simulink model "system_2022 [23-03-03]"  (R2022a)
settings: Solver=FixedStepAuto  StartTime=0.0  StopTime=30  FixedStep=0.05  MinStep=0.01  RelTol=1e-3  EnableMultiTasking=on
libraries: mbedblockslib x24, simulink x6, hdlsllib x6, slpidlib x3
(part 2 of 3)

== system system_2022 [23-03-03]/Subsystem/Pressure_Sensor_1/Pressure Conversion ==
  note: psi -> cmH2O
  note: Inspiration Pressure Calculation
      | Pg3 - Honeywell SPI Comms
  note: hex -> psi
  y : Inport
  Add : Sum
  Constant : Constant  Value=1638
  Constant1 : Constant  Value=120
  Constant2 : Constant  Value=13107
  Constant3 : Constant  Value=-60
  Constant4 : Constant  Value=1.01972
  Display : Display
  Display1 : Display
      settings: Format=hex (Stored Integer)
  Divide : Product  Inputs=*/
  Product : Product
  Product1 : Product
  Subtract : Sum  Inputs=+-
  Pressure : Outport
  wires:
  Constant/1 -> Subtract/2
  Subtract/1 -> Product/2
  Constant1/1 -> Product/1
  Product/1 -> Divide/1
  Constant2/1 -> Divide/2
  Constant3/1 -> Add/2
  Divide/1 -> Add/1
  Add/1 -> Product1/1
  Constant4/1 -> Product1/2
  Product1/1 -> Pressure/1, Display/1
  y/1 -> Display1/1, Subtract/1

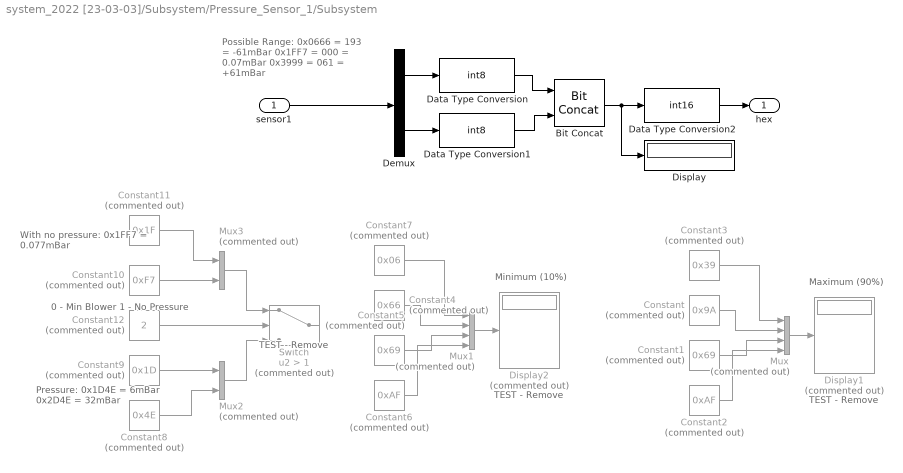
== system system_2022 [23-03-03]/Subsystem/Pressure_Sensor_1/Subsystem ==
  note: TEST - Remove
  note: 0 - Min Blower
      | 1 - No Pressure
  note: With no pressure:
      | 0x1FF7 = 0.077mBar
  note: Maximum (90%)
  note: Minimum (10%)
  note: Possible Range:
      | 0x0666 = 193 = -61mBar
      | 0x1FF7 = 000 = 0.07mBar
      | 0x3999 = 061 = +61mBar
  note: Pressure:
      | 0x1D4E = 6mBar
      | 0x2D4E = 32mBar
  note: TEST - Remove
  note: TEST - Remove
  sensor1 : Inport
  Bit Concat : hdlsllib/Logic and Bit Operations/Bit Concat  numInputs=2
  Constant : Constant  Commented=on  Value=0x9A
  Constant1 : Constant  Commented=on  Value=0x69
  Constant10 : Constant  Commented=on  Value=0xF7
  Constant11 : Constant  Commented=on  Value=0x1F
  Constant12 : Constant  Commented=on  Value=2
  Constant2 : Constant  Commented=on  Value=0xAF
  Constant3 : Constant  Commented=on  Value=0x39
  Constant4 : Constant  Commented=on  Value=0x66
  Constant5 : Constant  Commented=on  Value=0x69
  Constant6 : Constant  Commented=on  Value=0xAF
  Constant7 : Constant  Commented=on  Value=0x06
  Constant8 : Constant  Commented=on  Value=0x4E
  Constant9 : Constant  Commented=on  Value=0x1D
  Data Type Conversion : DataTypeConversion  OutDataTypeStr=int8  SaturateOnIntegerOverflow=off  RndMeth=Floor
  Data Type Conversion1 : DataTypeConversion  OutDataTypeStr=int8  SaturateOnIntegerOverflow=off  RndMeth=Floor
  Data Type Conversion2 : DataTypeConversion  OutDataTypeStr=int16  SaturateOnIntegerOverflow=off  RndMeth=Floor
  Demux : Demux  Outputs=2
  Display : Display
      settings: Format=hex (Stored Integer)
  Display1 : Display  Commented=on
      settings: Format=hex (Stored Integer)
  Display2 : Display  Commented=on
      settings: Format=hex (Stored Integer)
  Mux : Mux  Commented=on
  Mux1 : Mux  Commented=on
  Mux2 : Mux  Commented=on  Inputs=2
  Mux3 : Mux  Commented=on  Inputs=2
  Switch : Switch  Commented=on  Criteria=u2 > Threshold  Threshold=1  SaturateOnIntegerOverflow=off  InputSameDT=off
  hex : Outport
  wires:
  Constant3/1 -> Mux/1
  Constant/1 -> Mux/2
  Constant1/1 -> Mux/3
  Constant2/1 -> Mux/4
  Data Type Conversion/1 -> Bit Concat/1
  Data Type Conversion1/1 -> Bit Concat/2
  Demux/1 -> Data Type Conversion/1
  Demux/2 -> Data Type Conversion1/1
  Bit Concat/1 -> Display/1, Data Type Conversion2/1
  Mux/1 -> Display1/1
  Mux1/1 -> Display2/1
  Constant7/1 -> Mux1/1
  Constant6/1 -> Mux1/4
  Constant5/1 -> Mux1/3
  Constant4/1 -> Mux1/2
  Constant9/1 -> Mux2/1
  Constant8/1 -> Mux2/2
  Constant10/1 -> Mux3/2
  Constant11/1 -> Mux3/1
  Constant12/1 -> Switch/2
  Mux3/1 -> Switch/1
  Mux2/1 -> Switch/3
  Data Type Conversion2/1 -> hex/1
  sensor1/1 -> Demux/1

== system system_2022 [23-03-03]/Subsystem/Pressure_Sensor_1/Subsystem2 ==
  note: Need Global Array??
  note: Update single element of input array
  note: Extract Elements
  Array : Inport
  Index1 : Inport  Port=2
  Sense1 : Inport  Port=3
  Assignment : Assignment  IndexMode=Zero-based  DiagnosticForDimensions=Warning  IndexOptions=Index vector (port)  Indices=0  OutputSizes=1
  Out1 : Outport
  tag scope: PRES_AR1=global
  wires:
  Index1/1 -> Assignment/3
  Sense1/1 -> Assignment/2
  Assignment/1 -> [PRES_AR1], Out1/1
  Array/1 -> Assignment/1

== system system_2022 [23-03-03]/Subsystem/Pressure_Sensor_2/Pressure Conversion ==
  note: psi -> cmH2O
  note: Inspiration Pressure Calculation
      | Pg3 - Honeywell SPI Comms
  note: hex -> psi
  y : Inport
  Add : Sum
  Constant : Constant  Value=1638
  Constant1 : Constant  Value=120
  Constant2 : Constant  Value=13107
  Constant3 : Constant  Value=-60
  Constant4 : Constant  Value=1.01972
  Display : Display
  Display1 : Display
      settings: Format=hex (Stored Integer)
  Divide : Product  Inputs=*/
  Product : Product
  Product1 : Product
  Subtract : Sum  Inputs=+-
  Pressure : Outport
  wires:
  Constant/1 -> Subtract/2
  Subtract/1 -> Product/2
  Constant1/1 -> Product/1
  Product/1 -> Divide/1
  Constant2/1 -> Divide/2
  Constant3/1 -> Add/2
  Divide/1 -> Add/1
  Add/1 -> Product1/1
  Constant4/1 -> Product1/2
  Product1/1 -> Pressure/1, Display/1
  y/1 -> Display1/1, Subtract/1

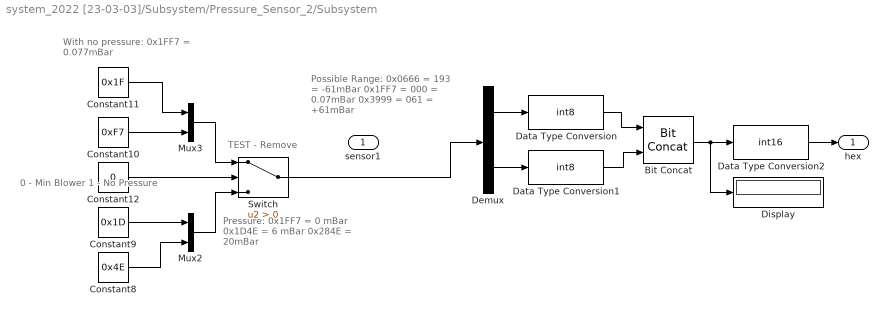
== system system_2022 [23-03-03]/Subsystem/Pressure_Sensor_2/Subsystem ==
  note: 0 - Min Blower
      | 1 - No Pressure
  note: With no pressure:
      | 0x1FF7 = 0.077mBar
  note: Possible Range:
      | 0x0666 = 193 = -61mBar
      | 0x1FF7 = 000 = 0.07mBar
      | 0x3999 = 061 = +61mBar
  note: Pressure:
      | 0x1FF7 = 0 mBar
      | 0x1D4E = 6 mBar
      | 0x284E = 20mBar
  note: TEST - Remove
  sensor1 : Inport
  Bit Concat : hdlsllib/Logic and Bit Operations/Bit Concat  numInputs=2
  Constant10 : Constant  Value=0xF7
  Constant11 : Constant  Value=0x1F
  Constant12 : Constant  Value=0
  Constant8 : Constant  Value=0x4E
  Constant9 : Constant  Value=0x1D
  Data Type Conversion : DataTypeConversion  OutDataTypeStr=int8  SaturateOnIntegerOverflow=off  RndMeth=Floor
  Data Type Conversion1 : DataTypeConversion  OutDataTypeStr=int8  SaturateOnIntegerOverflow=off  RndMeth=Floor
  Data Type Conversion2 : DataTypeConversion  OutDataTypeStr=int16  SaturateOnIntegerOverflow=off  RndMeth=Floor
  Demux : Demux  Outputs=2
  Display : Display
      settings: Format=hex (Stored Integer)
  Mux2 : Mux  Inputs=2
  Mux3 : Mux  Inputs=2
  Switch : Switch  Criteria=u2 > Threshold  SaturateOnIntegerOverflow=off  InputSameDT=off
  hex : Outport
  wires:
  Data Type Conversion/1 -> Bit Concat/1
  Data Type Conversion1/1 -> Bit Concat/2
  Demux/1 -> Data Type Conversion/1
  Demux/2 -> Data Type Conversion1/1
  Bit Concat/1 -> Display/1, Data Type Conversion2/1
  Constant9/1 -> Mux2/1
  Constant8/1 -> Mux2/2
  Constant10/1 -> Mux3/2
  Constant11/1 -> Mux3/1
  Constant12/1 -> Switch/2
  Mux3/1 -> Switch/1
  Mux2/1 -> Switch/3
  Switch/1 -> Demux/1
  Data Type Conversion2/1 -> hex/1

== system system_2022 [23-03-03]/Subsystem/Pressure_Sensor_2/Subsystem2 ==
  note: Update single element of input array
  note: Array "GoTo"
  Index1 : Inport
  Sense1 : Inport  Port=2
  Array : Inport  Port=3
  Assignment : Assignment  IndexMode=Zero-based  DiagnosticForDimensions=Warning  IndexOptions=Index vector (port)  Indices=0  OutputSizes=1
  Flow2 : Outport
  tag scope: PRES_AR2=global
  wires:
  Index1/1 -> Assignment/3
  Sense1/1 -> Assignment/2
  Assignment/1 -> [PRES_AR2], Flow2/1
  Array/1 -> Assignment/1

== system system_2022 [23-03-03]/Subsystem/Sensor_Monitor/Flow1_Monitor ==
  note: Exhale Flow Rate 1
      | Create Sub-System Status Commands
      | While inside threshold - Normal opertation (forward flow value)
      | If above/below threshold - Triggers alarm (alert value + alrm_trg)
  note: Alarm is triggered if Flow Rate is: [5 < Flow1 > 25] (SLM)
  note: Flow1 Trigger Values:
      | 0x41 = 65 - Normal Op
      | 0x42 = 66 - FlowRate2 High
      | 0x43 = 67 - FlowRate2 Low
  Flow1 : Inport
  Hi_Alert1 : Subsystem  TreatAsAtomicUnit=on
  If : If  IfExpression=(u1 <= 10)  ElseIfExpressions=(u1 >= 80)
  Lo_Alert1 : Subsystem  TreatAsAtomicUnit=on
  Merge : Merge  Inputs=3
  No_Alert1 : Subsystem  TreatAsAtomicUnit=on
  Fl1_Alrm : Outport
  wires:
  Flow1/1 -> If/1
  If/3 -> No_Alert1/Action
  No_Alert1/1(no_v) -> Merge/3
  Hi_Alert1/1(Out1) -> Merge/2
  Lo_Alert1/1(Out1) -> Merge/1
  If/2 -> Hi_Alert1/Action
  If/1 -> Lo_Alert1/Action
  Merge/1 -> Fl1_Alrm/1

== system system_2022 [23-03-03]/Subsystem/Sensor_Monitor/Flow2_Monitor ==
  note: Exhale Flow Rate 2
      | Create Sub-System Status Commands
      | While inside threshold - Normal opertation (forward flow value)
      | If above/below threshold - Triggers alarm (alert value + alrm_trg)
  note: Alarm is triggered if Flow Rate is: [5 < Flow1 > 25] (SLM)
  note: Flow1 Trigger Values:
      | 0x41 = 65 - Normal Op
      | 0x42 = 66 - FlowRate2 High
      | 0x43 = 67 - FlowRate2 Low
  Flow2 : Inport
  Hi_Alert2 : Subsystem  TreatAsAtomicUnit=on
  If : If  IfExpression=(u1 <= 10)  ElseIfExpressions=(u1 >= 80)
  Lo_Alert2 : Subsystem  TreatAsAtomicUnit=on
  Merge : Merge  Inputs=3
  No_Alert2 : Subsystem  TreatAsAtomicUnit=on
  Fl2_Alrm : Outport
  wires:
  Flow2/1 -> If/1
  If/3 -> No_Alert2/Action
  No_Alert2/1(no_v) -> Merge/3
  Hi_Alert2/1(Out1) -> Merge/2
  Lo_Alert2/1(Out1) -> Merge/1
  If/2 -> Hi_Alert2/Action
  If/1 -> Lo_Alert2/Action
  Merge/1 -> Fl2_Alrm/1

== system system_2022 [23-03-03]/Subsystem/Sensor_Monitor/Pressure1_Monitor ==
  note: Alarm is triggered if Pressure is: [5 < Prs > 25] (cmH20)
      | But Blower should also adjust pressure according to sensor reading.
  note: (Ex_Pressure)
      | Create Sub-System Status Commands
      | While inside threshold - Normal opertation (forward pressure value)
      | If above/below threshold - Triggers alarm (alert value + alrm_trg)
  Pr_I1 : Inport
  Display : Display
  Hi_Alert1 : Subsystem  TreatAsAtomicUnit=on
  If : If  IfExpression=(u1 <= 5)  ElseIfExpressions=(u1 >= 20)
  Lo_Alert1 : Subsystem  TreatAsAtomicUnit=on
  Merge : Merge  Inputs=3
  No_Alert1 : Subsystem  TreatAsAtomicUnit=on
  Pr1_Alrm : Outport
  wires:
  If/1 -> Lo_Alert1/Action
  If/3 -> No_Alert1/Action
  If/2 -> Hi_Alert1/Action
  Pr_I1/1 -> Display/1, If/1
  No_Alert1/1(no_v) -> Merge/3
  Lo_Alert1/1(Out1) -> Merge/1
  Hi_Alert1/1(Out1) -> Merge/2
  Merge/1 -> Pr1_Alrm/1

== system system_2022 [23-03-03]/Subsystem/Sensor_Monitor/Pressure2_Monitor ==
  note: Alarm is triggered if Pressure is: [5 < Prs > 25] (cmH20)
      | But Blower should also adjust pressure according to sensor reading.
  note: (Ex_Pressure)
      | Create Sub-System Status Commands
      | While inside threshold - Normal opertation (forward pressure value)
      | If above/below threshold - Triggers alarm (alert value + alrm_trg)
  Pr_E2 : Inport
  Display : Display
  Hi_Alert1 : Subsystem  TreatAsAtomicUnit=on
  If : If  IfExpression=(u1 <= 5)  ElseIfExpressions=(u1 >= 20)
  Lo_Alert1 : Subsystem  TreatAsAtomicUnit=on
  Merge : Merge  Inputs=3
  No_Alert1 : Subsystem  TreatAsAtomicUnit=on
  Pr2_Alrm : Outport
  wires:
  If/1 -> Lo_Alert1/Action
  If/3 -> No_Alert1/Action
  If/2 -> Hi_Alert1/Action
  Pr_E2/1 -> Display/1, If/1
  No_Alert1/1(no_v) -> Merge/3
  Lo_Alert1/1(Out1) -> Merge/1
  Hi_Alert1/1(Out1) -> Merge/2
  Merge/1 -> Pr2_Alrm/1

== system system_2022 [23-03-03]/Subsystem/Sensor_Monitor/Subsystem ==
  note: Alarm Hierarchy & Output
      | (Merge Sensor Alerts to single output)
  note: SIMULTANEOUS ALERTS?
      | -> Will Alert from Highest Priority
  note: Flow1_Alert
  note: Pres1_Alert
  note: Only 1 Alert Out
  note: Normal Value:
      | 0x31 (49) - Pressure1
      | 0x41 (65) - Flow1
      | 0x51 (81) - Pressure2
      | 0x61 (97) - Flow2
      | 0x71 (113) - FiO2
  note: Pres2_Alert
  note: Flow2_Alert
  note: FiO2_Alert
  note: ALARM Responses:
      | 0x21 - Normal Operation
      | 0x22 - Alarm Time_Out (2min)
      | 0x23 - Others ?
  Pr1_Alrm : Inport
  Fl1_Alrm : Inport  Port=2
  Pr2_Alrm : Inport  Port=3
  Fl2_Alrm : Inport  Port=4
  Fi_Alrm : Inport  Port=5
  FiO2_Alert : Subsystem  TreatAsAtomicUnit=on
  Flow_Alert1 : Subsystem  TreatAsAtomicUnit=on
  Flow_Alert2 : Subsystem  TreatAsAtomicUnit=on
  If : If  NumInputs=5  IfExpression=(u1 >= 50)  ElseIfExpressions=(u2 >= 66), (u3 >= 82), (u4 >= 98), (u5 >= 114)  ZeroCross=off
  Merge : Merge  Inputs=6
  No_Alert : Subsystem  TreatAsAtomicUnit=on
  Press_Alert1 : Subsystem  TreatAsAtomicUnit=on
  Press_Alert2 : Subsystem  TreatAsAtomicUnit=on
  ALRM_Out : Outport
  wires:
  If/6 -> No_Alert/Action
  Merge/1 -> ALRM_Out/1
  Pr2_Alrm/1 -> Press_Alert2/1(P2_Alrm), If/3
  Fl2_Alrm/1 -> Flow_Alert2/1(F2_Alrm), If/4
  Fi_Alrm/1 -> FiO2_Alert/1(FiO2_Alrm), If/5
  If/3 -> Press_Alert2/Action
  If/4 -> Flow_Alert2/Action
  If/5 -> FiO2_Alert/Action
  Press_Alert2/1(Out1) -> Merge/3
  Flow_Alert2/1(Out1) -> Merge/4
  FiO2_Alert/1(Out1) -> Merge/5
  No_Alert/1(Out1) -> Merge/6
  Fl1_Alrm/1 -> Flow_Alert1/1(F1_Alrm), If/2
  Pr1_Alrm/1 -> Press_Alert1/1(P1_Alrm), If/1
  If/2 -> Flow_Alert1/Action
  If/1 -> Press_Alert1/Action
  Flow_Alert1/1(Out1) -> Merge/2
  Press_Alert1/1(Out1) -> Merge/1

== system system_2022 [23-03-03]/Subsystem/Sub-Systems Read/HMI_Test_Input ==
  Dummy Startup : Stateflow chart  TreatAsAtomicUnit=on
  HMI Graph Test : Stateflow chart  TreatAsAtomicUnit=on
  Reshape : Reshape  OutputDimensionality=Column vector (2-D)
  H_Cmd : Outport
  wires:
  Reshape/1 -> H_Cmd/1
  HMI Graph Test/1(output) -> Reshape/1

== system system_2022 [23-03-03]/Subsystem/Sub-Systems Write/Combine All ==
  note: 51 = 0x33 = No Alarm
      | 33 = 0x21 = No Alarm
  note: Select highest priority Alert & Update to HMI Array
  note: Write 5 byte array to HMI
      | + 1 Alarm byte
  note: Output Highest Priority
      | 1st - SubSystem
      | 2nd - Sensors
  HMI : Inport
  AlmSBS : Inport  Port=2
  AlmSNS : Inport  Port=3
  Constant2 : Constant  Value=5
  Display : Display
  Display1 : Display
  Display2 : Display
  Hi_Alert1 : Subsystem  TreatAsAtomicUnit=on
  Hi_Alert2 : Subsystem  TreatAsAtomicUnit=on
  If : If  NumInputs=2  IfExpression=(u1 > 33)  ElseIfExpressions=(u2 >= 20)
  Lo_Alert1 : Subsystem  TreatAsAtomicUnit=on
  Merge : Merge  Inputs=3
  Subsystem3 : Subsystem
  Alarm : Outport
  HMI_Array : Outport  Port=2
  wires:
  HMI/1 -> Subsystem3/3(Array)
  Constant2/1 -> Subsystem3/1(Index1)
  Subsystem3/1(Flow2) -> HMI_Array/1
  If/2 -> Hi_Alert1/Action
  If/1 -> Lo_Alert1/Action
  AlmSBS/1 -> Display/1, Lo_Alert1/1(AlmSBS), If/1
  AlmSNS/1 -> Display1/1, Hi_Alert1/1(AlmSNS), If/2
  Hi_Alert1/1(Out1) -> Merge/2
  Lo_Alert1/1(Out1) -> Merge/1
  Merge/1 -> Subsystem3/2(Sense1), Display2/1, Alarm/1
  If/3 -> Hi_Alert2/Action
  Hi_Alert2/1(Out1) -> Merge/3

== system system_2022 [23-03-03]/Subsystem/System Update and Heirarchy/Alarm Priority ==
  note: Create final ALARM message
  note: What if BOTH ? - consecutive
  note: Single byte Alert:
      | UPPER 4-bits:
      | 0x10 - Power
      | 0x20 - Alarm
      | 0x30 - Pressure
      | 0x40 - Flow...
      |
      | LOWER 4-bits:
      | over/under/bat_%/time_out
  note: Remove this whole block and forward Alarm Codes directly
  note: Alarm Alerts:
      | 0x21 - No Alarm
      | 0x22 - Over_Time
  note: PSU Alerts:
      | 0x11 - Normal (AC)
      | 0x12 - Battery 75%
      | 0x13 - Battery 50%
      | 0x14 - Battery 25%
  P_Alrm : Inport
  A_Alrm : Inport  Port=2
  Alarm Alert : Subsystem  TreatAsAtomicUnit=on
  Data Type Conversion : DataTypeConversion  OutDataTypeStr=double  SaturateOnIntegerOverflow=off  RndMeth=Floor
  Display2 : Display
  If : If  NumInputs=2  IfExpression=(u1 > 17)  ElseIfExpressions=(u2 > 33)
  Merge : Merge  Inputs=3
  No_Alarm1 : Subsystem  TreatAsAtomicUnit=on
  Power Alert : Subsystem  TreatAsAtomicUnit=on
  ALRM_Out : Outport
  wires:
  P_Alrm/1 -> Data Type Conversion/1, If/1
  A_Alrm/1 -> If/2
  If/1 -> Power Alert/Action
  Merge/1 -> Display2/1, ALRM_Out/1
  Power Alert/1(Out1) -> Merge/1
  Alarm Alert/1(Out1) -> Merge/2
  No_Alarm1/1(Out1) -> Merge/3
  Data Type Conversion/1 -> Power Alert/1(P_Alrm)
  If/2 -> Alarm Alert/Action
  If/3 -> No_Alarm1/Action

== system system_2022 [23-03-03]/Subsystem/System Update and Heirarchy/Get Value and Array Index ==
  note: Get byte[0]
  note: Extract Specific Byte from HMI_Input Array
  note: Get byte[1]
  Usr_In : Inport
  Constant1 : Constant  OutDataTypeStr=uint8
  Constant2 : Constant  Value=0  OutDataTypeStr=uint8
  Display1 : Display
  Display12 : Display
  Display4 : Display
  Index Vector : MultiPortSwitch  DataPortOrder=Zero-based contiguous  Inputs=1  zeroidx=on  OutDataTypeStr=uint8  SaturateOnIntegerOverflow=off  InputSameDT=off
  Index Vector1 : MultiPortSwitch  DataPortOrder=Zero-based contiguous  Inputs=1  zeroidx=on  OutDataTypeStr=uint8  SaturateOnIntegerOverflow=off  InputSameDT=off
  HMI_Cmd1 : Outport
  New_Val1 : Outport  Port=2
  wires:
  Index Vector/1 -> HMI_Cmd1/1, Display4/1
  Constant2/1 -> Index Vector/1
  Usr_In/1 -> Display12/1, Index Vector1/2, Index Vector/2
  Constant1/1 -> Index Vector1/1
  Index Vector1/1 -> Display1/1, New_Val1/1

== system system_2022 [23-03-03]/Subsystem/System Update and Heirarchy/Initial IPAP EPAP ==
  note: [1x2] to [2x1]
  note: Initial IPAP & EPAP Values:
      | (only on boot-up)
  H_Cmd : Inport
  Chart : Stateflow chart  TreatAsAtomicUnit=on
      settings: PortSchema="{\"entries\":[{\"content\":{\"sides\":[{\"content\":{\"connectorIds\":[]},\"type\":\"ConnectorPlacement.EquallySpacedRectSide\",\"uuid\":\"6628deca-e0b8-40ca-949f-ac0e837bdfd6\"},{\"content\":{\"connectorIds\":[\"Out2\",\"Out1\"],\"side\":\"RIGHT\"},\"type\":\"ConnectorPlacement.EquallySpacedRectSide\",\"uuid\":\"942c872d-7aee-48e1-8ef8-861eef53b55a\"},{\"content\":{\"connectorIds\":[],\"side\":\"TOP\"},\"type\":\"ConnectorPlacement.EquallySpacedRectSide\",\"uuid\":\"7d4bff24-2b40-487e-be4f-fa01986134b0\"}]},\"type\":\"ConnectorPlacement.EquallySpacedConnector\",\"uuid\":\"61848f08-0c78-4d83-a956-79c751d6cd3c\"}],\"packageUris\":[\"http://schema.mathworks.com/mf0/Connector/R2020b\"],\"version\":\"1.0\"}"
  Display : Display
  If : If  IfExpression=u1 > 4
  If Action Subsystem : Subsystem  TreatAsAtomicUnit=on
  If Action Subsystem1 : Subsystem  TreatAsAtomicUnit=on
  Merge : Merge
  Reshape : Reshape  OutputDimensionality=Column vector (2-D)
  output : Outport
  wires:
  Merge/1 -> Display/1, output/1
  If Action Subsystem1/1(Out1) -> Merge/2
  If/1 -> If Action Subsystem1/Action
  If/2 -> If Action Subsystem/Action
  Chart/2(nope) -> If/1
  H_Cmd/1 -> If Action Subsystem1/1(output)
  If Action Subsystem/1(Out1) -> Merge/1
  Chart/1(output) -> Reshape/1
  Reshape/1 -> If Action Subsystem/1(output)

== system system_2022 [23-03-03]/Subsystem/System Update and Heirarchy/Power_CMD ==
  note: REMOVED PSU CHECK (ALARM & HMI WILL CHECK)
  note: PASS PSU CODE DIRECTLY
  note: 0x14 = 20dec
  note: (PSU)
      | Read Sub-System Status Commands
      | Normal operation = No 2nd byte
      | Event trigger (2) = DC voltage forwarded
  note: Get Lower 4 bits
  note: Battery Status:
      | 0x10 - AC
      | 0x11 - 75%
      | 0x12 - 50%
      | 0x13 - 25%
  note: PSU Alerts:
      | 0x11 - Normal (AC)
      | 0x12 - Battery 75%
      | 0x13 - Battery 50%
      | 0x14 - Battery 25%
  note: Error Code (99)
  P_Cmd : Inport
  AC POWER : Subsystem  Commented=on  TreatAsAtomicUnit=on
  Bitwise Operator1 : simulink/Logic and Bit Operations/Bitwise Operator  Commented=on  logicop=AND  UseBitMask=on  BitMask=bin2dec('00001111')  BitMaskRealWorld=Stored Integer
  Constant : Constant  Commented=on  Value=0x13
  Constant2 : Constant  Commented=on  Value=0x14  SampleTime=-1
  Constant3 : Constant  Commented=on  Value=0x63  SampleTime=-1
  DC POWER : Subsystem  Commented=on  TreatAsAtomicUnit=on
  Display1 : Display  Commented=on
      settings: Format=hex (Stored Integer)
  ERROR MSG1 : Subsystem  Commented=on  TreatAsAtomicUnit=on
  Merge1 : Merge  Commented=on  Inputs=4
  Power_Other : Subsystem  Commented=on  TreatAsAtomicUnit=on
  Switch Case1 : SwitchCase  Commented=on  CaseConditions={0x01, 0x02, 0x03}
  P_Alrm : Outport
  wires:
  Switch Case1/4 -> ERROR MSG1/Action
  Constant2/1 -> Power_Other/1(In1)
  Switch Case1/1 -> AC POWER/Action
  Switch Case1/3 -> Power_Other/Action
  Bitwise Operator1/1 -> Switch Case1/1
  Switch Case1/2 -> DC POWER/Action
  Constant3/1 -> ERROR MSG1/1(In1)
  Power_Other/1(Out1) -> Merge1/3
  ERROR MSG1/1(Out1) -> Merge1/4
  AC POWER/1(Out1) -> Merge1/1
  DC POWER/1(DC_out) -> Merge1/2
  P_Cmd/1 -> P_Alrm/1
  Constant/1 -> DC POWER/1(DC_in), Bitwise Operator1/1
  Merge1/1 -> Display1/1

== system system_2022 [23-03-03]/Subsystem/System Update and Heirarchy/Update Internal Variables ==
  note: Remove Var_Arr:
      | Unless used internally?
  note: Update the system variable with User_Input
      | Save new value to correct Array element for system update
  note: Variables:
      | [0] - CPAP
      | [1] - EPAP
      | [2] - IPAP
      | [3] - FiO2
      | [4] - APNEA
      | [5] - Mode
  note: Array Element
  note: Value to be stored
  note: Should be from updated HMI
      | Input Value Array[0-4] .
      | Single value at the moment.
  note: HMI - INPUTS:
      | 0x03 (03) - CPAP
      | 0x13 (19) - EPAP
      | 0x23 (35) - IPAP
      | 0x33 (51) - FiO2
      | 0x43 (67) - APNEA
  note: Other Inputs:
      | 0x11 (17) - Start
      | 0x19 (25) - Mode
  HMI_Cmd1 : Inport
  New_Val1 : Inport  Port=2
  Display : Display
  Display1 : Display
  Display2 : Display
  Get_HMI_Values : Subsystem
  HMI_CMD1 : Subsystem
  wires:
  HMI_CMD1/1(Element1) -> Get_HMI_Values/1(Element1), Display/1
  HMI_Cmd1/1 -> HMI_CMD1/1(H_Cmd)
  Get_HMI_Values/1(Var_Arr) -> Display2/1
  New_Val1/1 -> Get_HMI_Values/2(Value1), Display1/1

== system system_2022 [23-03-03]/Subsystem/Sensor_Monitor/Flow1_Monitor/Hi_Alert1 ==
  note: If within normal pressure range,
      | forward that value to HMI for display
  note: Above FlowRate threshold = 0x42
  note: 0x42 = 66 dec
  note: Above Flow Rate (1) Threshold
  Action Port : ActionPort  ActionPortLabel=elseif((u1 >= 80))
  Alert1 : Constant  Value=66
  Out1 : Outport
  wires:
  Alert1/1 -> Out1/1

== system system_2022 [23-03-03]/Subsystem/Sensor_Monitor/Flow1_Monitor/Lo_Alert1 ==
  note: Below Flow Rate (1) Threshold
  note: Below FlowRate Threshold = 0x43
  note: 0x43 = 67 dec
  Action Port : ActionPort  ActionPortLabel=if((u1 <= 10))
  Alert1 : Constant  Value=67
  Out1 : Outport
  wires:
  Alert1/1 -> Out1/1

== system system_2022 [23-03-03]/Subsystem/Sensor_Monitor/Flow1_Monitor/No_Alert1 ==
  note: No Alert (normal range) = 0x01
  note: 0x41 = 65 dec
  note: Within Flow Rate (1) Threshold
  Action Port : ActionPort  ActionPortLabel=else
  Alert1 : Constant  Value=65
  no_v : Outport
  wires:
  Alert1/1 -> no_v/1

== system system_2022 [23-03-03]/Subsystem/Sensor_Monitor/Flow2_Monitor/Hi_Alert2 ==
  note: If within normal pressure range,
      | forward that value to HMI for display
  note: Above FlowRate threshold = 0x42
  note: 0x62 = 98 dec
  note: Below Flow Rate (2) Threshold
  Action Port : ActionPort  ActionPortLabel=elseif((u1 >= 80))
  Alert1 : Constant  Value=98
  Out1 : Outport
  wires:
  Alert1/1 -> Out1/1

== system system_2022 [23-03-03]/Subsystem/Sensor_Monitor/Flow2_Monitor/Lo_Alert2 ==
  note: Below Flow Rate (2) Threshold
  note: Below FlowRate Threshold = 0x43
  note: 0x63 = 99 dec
  Action Port : ActionPort  ActionPortLabel=if((u1 <= 10))
  Alert1 : Constant  Value=99
  Out1 : Outport
  wires:
  Alert1/1 -> Out1/1

== system system_2022 [23-03-03]/Subsystem/Sensor_Monitor/Flow2_Monitor/No_Alert2 ==
  note: No Alert (normal range) = 0x01
  note: 0x61 = 97 dec
  note: Within Flow Rate (2) Threshold
  Action Port : ActionPort  ActionPortLabel=else
  Alert1 : Constant  Value=97
  no_v : Outport
  wires:
  Alert1/1 -> no_v/1

== system system_2022 [23-03-03]/Subsystem/Sensor_Monitor/Pressure1_Monitor/Hi_Alert1 ==
  note: Above Pressure threshold
  note: 0x32 = 50 dec
  note: Above Pressure Threshold = 0x32
  Action Port : ActionPort  ActionPortLabel=elseif((u1 >= 20))
  Alert1 : Constant  Value=50
  Out1 : Outport
  wires:
  Alert1/1 -> Out1/1

== system system_2022 [23-03-03]/Subsystem/Sensor_Monitor/Pressure1_Monitor/Lo_Alert1 ==
  note: 0x33 = 51 dec
  note: Below Pressure Threshold = 0x33
  Action Port : ActionPort  ActionPortLabel=if((u1 <= 5))
  Alert1 : Constant  Value=51
  Out1 : Outport
  wires:
  Alert1/1 -> Out1/1

== system system_2022 [23-03-03]/Subsystem/Sensor_Monitor/Pressure1_Monitor/No_Alert1 ==
  note: No Trigger - Within Range
  note: No Alert (normal range)
  note: If within normal pressure range,
      | forward that value to HMI for display
  note: 0x31 - 49 dec
  Action Port : ActionPort  ActionPortLabel=else
  Alert1 : Constant  Value=49
  no_v : Outport
  wires:
  Alert1/1 -> no_v/1

== system system_2022 [23-03-03]/Subsystem/Sensor_Monitor/Pressure2_Monitor/Hi_Alert1 ==
  note: Above Pressure threshold
  note: 0x52 = 82 dec
  note: Above Pressure (2) Threshold = 0x52
  Action Port : ActionPort  ActionPortLabel=elseif((u1 >= 20))
  Alert1 : Constant  Value=82
  Out1 : Outport
  wires:
  Alert1/1 -> Out1/1

== system system_2022 [23-03-03]/Subsystem/Sensor_Monitor/Pressure2_Monitor/Lo_Alert1 ==
  note: 0x53 = 83 dec
  note: Below Pressure (2) Threshold = 0x53
  Action Port : ActionPort  ActionPortLabel=if((u1 <= 5))
  Alert1 : Constant  Value=83
  Out1 : Outport
  wires:
  Alert1/1 -> Out1/1

== system system_2022 [23-03-03]/Subsystem/Sensor_Monitor/Pressure2_Monitor/No_Alert1 ==
  note: No Trigger - Within Range
  note: No Alert (normal range)
  note: If within normal pressure range,
      | forward that value to HMI for display
  note: 0x31 - 49 dec
  Action Port : ActionPort  ActionPortLabel=else
  Alert1 : Constant  Value=49
  no_v : Outport
  wires:
  Alert1/1 -> no_v/1

== system system_2022 [23-03-03]/Subsystem/Sensor_Monitor/Subsystem/FiO2_Alert ==
  note: Pressure Alert
  FiO2_Alrm : Inport
  Action Port : ActionPort  ActionPortLabel=elseif( (u5 >= 114))
  Out1 : Outport
  wires:
  FiO2_Alrm/1 -> Out1/1

== system system_2022 [23-03-03]/Subsystem/Sensor_Monitor/Subsystem/Flow_Alert1 ==
  note: Either Pressure OR Power Alert!
  F1_Alrm : Inport
  Action Port : ActionPort  ActionPortLabel=elseif((u2 >= 66))
  Out1 : Outport
  wires:
  F1_Alrm/1 -> Out1/1

== system system_2022 [23-03-03]/Subsystem/Sensor_Monitor/Subsystem/Flow_Alert2 ==
  note: Pressure Alert
  F2_Alrm : Inport
  Action Port : ActionPort  ActionPortLabel=elseif( (u4 >= 98))
  Out1 : Outport
  wires:
  F2_Alrm/1 -> Out1/1

== system system_2022 [23-03-03]/Subsystem/Sensor_Monitor/Subsystem/No_Alert ==
  note: 0X01 = NO ALERTS
  note: Normal Opertaion (No Alerts)
  Action Port : ActionPort  ActionPortLabel=else
  Constant : Constant  Value=33
  Out1 : Outport
  wires:
  Constant/1 -> Out1/1

== system system_2022 [23-03-03]/Subsystem/Sensor_Monitor/Subsystem/Press_Alert1 ==
  note: Pressure Alert
  P1_Alrm : Inport
  Action Port : ActionPort  ActionPortLabel=if((u1 >= 50))
  Out1 : Outport
  wires:
  P1_Alrm/1 -> Out1/1

== system system_2022 [23-03-03]/Subsystem/Sensor_Monitor/Subsystem/Press_Alert2 ==
  note: Pressure (2) High or Low
  P2_Alrm : Inport
  Action Port : ActionPort  ActionPortLabel=elseif( (u3 >= 82))
  Out1 : Outport
  wires:
  P2_Alrm/1 -> Out1/1

== system system_2022 [23-03-03]/Subsystem/Sub-Systems Write/Combine All/Hi_Alert1 ==
  note: Sensor Alerts Take Lowest Priority
  AlmSNS : Inport
  Action Port : ActionPort  ActionPortLabel=elseif((u2 >= 20))
  Out1 : Outport
  wires:
  AlmSNS/1 -> Out1/1

== system system_2022 [23-03-03]/Subsystem/Sub-Systems Write/Combine All/Hi_Alert2 ==
  note: 0x21 = 33 dec
  note: If No Alert
  Action Port : ActionPort  ActionPortLabel=else
  No Alert1 : Constant  Value=33
  Out1 : Outport
  wires:
  No Alert1/1 -> Out1/1

== system system_2022 [23-03-03]/Subsystem/Sub-Systems Write/Combine All/Lo_Alert1 ==
  note: Sub-System Alert Take Highest Priority
  AlmSBS : Inport
  Action Port : ActionPort  ActionPortLabel=if((u1 > 33))
  Out1 : Outport
  wires:
  AlmSBS/1 -> Out1/1

== system system_2022 [23-03-03]/Subsystem/Sub-Systems Write/Combine All/Subsystem3 ==
  note: Need Global Array??
  note: Update single element of input array
  Index1 : Inport
  Sense1 : Inport  Port=2
  Array : Inport  Port=3
  Assignment : Assignment  IndexMode=Zero-based  DiagnosticForDimensions=Warning  IndexOptions=Index vector (port)  Indices=0  OutputSizes=1
  Flow2 : Outport
  wires:
  Index1/1 -> Assignment/3
  Sense1/1 -> Assignment/2
  Assignment/1 -> Flow2/1
  Array/1 -> Assignment/1

== system system_2022 [23-03-03]/Subsystem/System Update and Heirarchy/Alarm Priority/Alarm Alert ==
  note: 0x22 = 34 dec
  note: ALARM OVER 2 MINUTES
  Action Port : ActionPort  ActionPortLabel=elseif((u2 > 33))
  Constant : Constant  Value=34
  Out1 : Outport
  wires:
  Constant/1 -> Out1/1

== system system_2022 [23-03-03]/Subsystem/System Update and Heirarchy/Alarm Priority/No_Alarm1 ==
  note: 0x11 = Normal Operation
  note: Normal Opertaion (No Alerts)
  Action Port : ActionPort  ActionPortLabel=else
  Constant : Constant  Value=33
  Out1 : Outport
  wires:
  Constant/1 -> Out1/1

== system system_2022 [23-03-03]/Subsystem/System Update and Heirarchy/Alarm Priority/Power Alert ==
  note: Battery Alert & Capacity in same byte
  note: PSU Power Alert + Battery %
  P_Alrm : Inport
  Action Port : ActionPort  ActionPortLabel=if((u1 > 17))
  Out1 : Outport
  wires:
  P_Alrm/1 -> Out1/1

== system system_2022 [23-03-03]/Subsystem/System Update and Heirarchy/Initial IPAP EPAP/If Action Subsystem ==
  output : Inport
  Action Port : ActionPort  ActionPortLabel=else
  Out1 : Outport
  wires:
  output/1 -> Out1/1

== system system_2022 [23-03-03]/Subsystem/System Update and Heirarchy/Initial IPAP EPAP/If Action Subsystem1 ==
  output : Inport
  Action Port : ActionPort  ActionPortLabel=if(u1 > 4)
  Out1 : Outport
  wires:
  output/1 -> Out1/1

== system system_2022 [23-03-03]/Subsystem/System Update and Heirarchy/Power_CMD/AC POWER ==
  Action Port : ActionPort
  Constant : Constant  Value=0x10
  Out1 : Outport
  wires:
  Constant/1 -> Out1/1

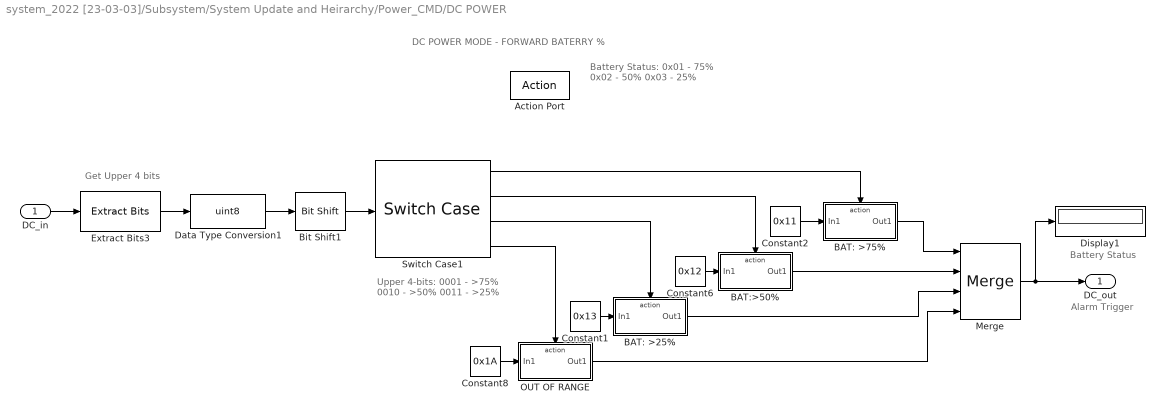
== system system_2022 [23-03-03]/Subsystem/System Update and Heirarchy/Power_CMD/DC POWER ==
  note: Battery Status
  note: Upper 4-bits:
      | 0001 - >75%
      | 0010 - >50%
      | 0011 - >25%
  note: DC POWER MODE - FORWARD BATERRY %
  note: Get Upper 4 bits
  note: Alarm Trigger
  note: Battery Status:
      | 0x01 - 75%
      | 0x02 - 50%
      | 0x03 - 25%
  DC_in : Inport
  Action Port : ActionPort
  BAT: >25% : Subsystem  TreatAsAtomicUnit=on
  BAT: >75% : Subsystem  TreatAsAtomicUnit=on
  BAT:>50% : Subsystem  TreatAsAtomicUnit=on
  Bit Shift1 : hdlsllib/Logic and Bit Operations/Bit Shift  mode=Shift Right Logical  N=4
  Constant1 : Constant  Value=0x13  SampleTime=-1
  Constant2 : Constant  Value=0x11  SampleTime=-1
  Constant6 : Constant  Value=0x12  SampleTime=-1
  Constant8 : Constant  Value=0x1A  SampleTime=-1
  Data Type Conversion1 : DataTypeConversion  OutDataTypeStr=uint8  SaturateOnIntegerOverflow=off  RndMeth=Floor
  Display1 : Display
      settings: Format=hex (Stored Integer)
  Extract Bits3 : simulink/Logic and Bit Operations/Extract Bits  bitsToExtract=Upper half  numBits=8  bitIdxRange=[0 7]  outScalingMode=Preserve fixed-point scaling
  Merge : Merge  Inputs=4
  OUT OF RANGE : Subsystem  TreatAsAtomicUnit=on
  Switch Case1 : SwitchCase  CaseConditions={0x01, 0x02, 0x03}
  DC_out : Outport
  wires:
  Switch Case1/3 -> BAT: >25%/Action
  Merge/1 -> DC_out/1, Display1/1
  Constant8/1 -> OUT OF RANGE/1(In1)
  OUT OF RANGE/1(Out1) -> Merge/4
  BAT: >75%/1(Out1) -> Merge/1
  Extract Bits3/1 -> Data Type Conversion1/1
  Switch Case1/2 -> BAT:>50%/Action
  Bit Shift1/1 -> Switch Case1/1
  BAT:>50%/1(Out1) -> Merge/2
  Constant6/1 -> BAT:>50%/1(In1)
  Data Type Conversion1/1 -> Bit Shift1/1
  BAT: >25%/1(Out1) -> Merge/3
  Switch Case1/4 -> OUT OF RANGE/Action
  Switch Case1/1 -> BAT: >75%/Action
  Constant2/1 -> BAT: >75%/1(In1)
  Constant1/1 -> BAT: >25%/1(In1)
  DC_in/1 -> Extract Bits3/1

== system system_2022 [23-03-03]/Subsystem/System Update and Heirarchy/Power_CMD/ERROR MSG1 ==
  In1 : Inport
  Action Port : ActionPort
  Out1 : Outport
  wires:
  In1/1 -> Out1/1

== system system_2022 [23-03-03]/Subsystem/System Update and Heirarchy/Power_CMD/Power_Other ==
  note: Do what with each
      | Triggerd bit?
  In1 : Inport
  Action Port : ActionPort
  Out1 : Outport
  wires:
  In1/1 -> Out1/1

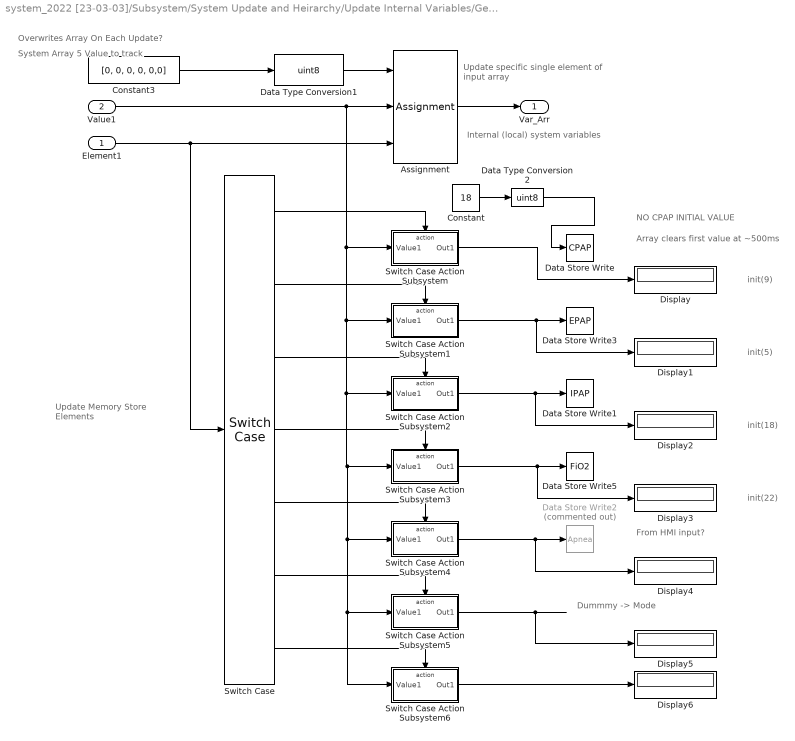
== system system_2022 [23-03-03]/Subsystem/System Update and Heirarchy/Update Internal Variables/Get_HMI_Values ==
  note: init(18)
  note: NO CPAP INITIAL VALUE
  note: Internal (local) system variables
  note: System Array
      | 5 Value to track
  note: Update specific single
      | element of input array
  note: Overwrites Array On Each Update?
  note: Update Memory
      | Store Elements
  note: From HMI input?
  note: init(5)
  note: init(9)
  note: init(22)
  note: Array clears first value at ~500ms
  note: Dummmy -> Mode
  Element1 : Inport
  Value1 : Inport  Port=2
  Assignment : Assignment  IndexMode=Zero-based  DiagnosticForDimensions=Warning  IndexOptions=Index vector (port)  Indices=0  OutputSizes=1
  Constant : Constant  Value=18
  Constant3 : Constant  Value=[0, 0, 0, 0, 0,0]
  Data Store Write : DataStoreWrite  DataStoreName=CPAP  IndexOptions=Index vector (dialog)  Indices=1  OutputSizes=1
  Data Store Write1 : DataStoreWrite  DataStoreName=IPAP  DataStoreElements=IPAP  IndexOptions=Index vector (dialog)  Indices=1  OutputSizes=1
  Data Store Write2 : DataStoreWrite  Commented=on  DataStoreName=Apnea  IndexOptions=Index vector (dialog)  Indices=1  OutputSizes=1
  Data Store Write3 : DataStoreWrite  DataStoreName=EPAP  DataStoreElements=EPAP  IndexOptions=Index vector (dialog)  Indices=1  OutputSizes=1
  Data Store Write5 : DataStoreWrite  DataStoreName=FiO2  IndexOptions=Index vector (dialog)  Indices=1  OutputSizes=1
  Data Type Conversion1 : DataTypeConversion  OutDataTypeStr=uint8  SaturateOnIntegerOverflow=off  RndMeth=Floor
  Data Type Conversion2 : DataTypeConversion  OutDataTypeStr=uint8  SaturateOnIntegerOverflow=off  RndMeth=Floor
  Display{,1..6} (7 alike) : Display
  Switch Case : SwitchCase  CaseConditions={0,1,2,3,4,5}
  Switch Case Action Subsystem : Subsystem  TreatAsAtomicUnit=on
  Switch Case Action Subsystem1 : Subsystem  TreatAsAtomicUnit=on
  Switch Case Action Subsystem2 : Subsystem  TreatAsAtomicUnit=on
  Switch Case Action Subsystem3 : Subsystem  TreatAsAtomicUnit=on
  Switch Case Action Subsystem4 : Subsystem  TreatAsAtomicUnit=on
  Switch Case Action Subsystem5 : Subsystem  TreatAsAtomicUnit=on
  Switch Case Action Subsystem6 : Subsystem  TreatAsAtomicUnit=on
  Var_Arr : Outport
  wires:
  Element1/1 -> Assignment/3, Switch Case/1
  Switch Case Action Subsystem3/1(Out1) -> Data Store Write5/1, Display3/1
  Switch Case Action Subsystem4/1(Out1) -> Data Store Write2/1, Display4/1
  Switch Case Action Subsystem6/1(Out1) -> Display6/1
  Switch Case Action Subsystem2/1(Out1) -> Data Store Write1/1, Display2/1
  Value1/1 -> Switch Case Action Subsystem1/1(Value1), Switch Case Action Subsystem2/1(Value1), Switch Case Action Subsystem5/1(Value1), Switch Case Action Subsystem6/1(Value1), Switch Case Action Subsystem4/1(Value1), Switch Case Action Subsystem3/1(Value1), Switch Case Action Subsystem/1(Value1), Assignment/2
  Switch Case Action Subsystem1/1(Out1) -> Data Store Write3/1, Display1/1
  Constant3/1 -> Data Type Conversion1/1
  Switch Case Action Subsystem/1(Out1) -> Display/1
  Assignment/1 -> Var_Arr/1
  Data Type Conversion1/1 -> Assignment/1
  Switch Case Action Subsystem5/1(Out1) -> Display5/1
  Switch Case/1 -> Switch Case Action Subsystem/Action
  Switch Case/2 -> Switch Case Action Subsystem1/Action
  Switch Case/3 -> Switch Case Action Subsystem2/Action
  Switch Case/4 -> Switch Case Action Subsystem3/Action
  Switch Case/5 -> Switch Case Action Subsystem4/Action
  Switch Case/6 -> Switch Case Action Subsystem5/Action
  Switch Case/7 -> Switch Case Action Subsystem6/Action
  Constant/1 -> Data Type Conversion2/1
  Data Type Conversion2/1 -> Data Store Write/1

== system system_2022 [23-03-03]/Subsystem/System Update and Heirarchy/Update Internal Variables/HMI_CMD1 ==
  note: was arr[5]
  note: (HMI)
      | Read Sub-System Status Commands
  note: Get Lower 4 bits
  note: MSG (lower):
      | 0x01 - Start/Stop
      | 0x03 - User Input
      | 0x05 - Alarm Silence
      | 0x09 - Mode
  H_Cmd : Inport
  Alarm : Subsystem  TreatAsAtomicUnit=on
  Bitwise Operator : simulink/Logic and Bit Operations/Bitwise Operator  logicop=AND  UseBitMask=on  BitMask=bin2dec('00001111')  BitMaskRealWorld=Stored Integer
  Constant5 : Constant  Value=0
  Display : Display
  Display1 : Display
  ERROR MSG : Subsystem  TreatAsAtomicUnit=on
  MODE : Subsystem  TreatAsAtomicUnit=on
  Merge2 : Merge  Inputs=5
  START : Subsystem  TreatAsAtomicUnit=on
  Switch Case : SwitchCase  CaseConditions={0x01, 0x03, 0x05, 0x09}
  User_Input : Subsystem  TreatAsAtomicUnit=on
  Element1 : Outport
  wires:
  Constant5/1 -> ERROR MSG/1(In1)
  Bitwise Operator/1 -> Display1/1, Switch Case/1
  Switch Case/5 -> ERROR MSG/Action
  Merge2/1 -> Element1/1
  H_Cmd/1 -> Display/1, START/1(H_Cmd), User_Input/1(H_Cmd), Alarm/1(H_Cmd), MODE/1(H_Cmd), Bitwise Operator/1
  Switch Case/1 -> START/Action
  Switch Case/2 -> User_Input/Action
  Switch Case/3 -> Alarm/Action
  Switch Case/4 -> MODE/Action
  START/1(Elem) -> Merge2/1
  User_Input/1(Arr1) -> Merge2/2
  Alarm/1(Elem) -> Merge2/3
  MODE/1(Elem) -> Merge2/4
  ERROR MSG/1(Out1) -> Merge2/5

== system system_2022 [23-03-03]/Subsystem/System Update and Heirarchy/Power_CMD/DC POWER/BAT: >25% ==
  In1 : Inport
  Action Port : ActionPort
  Out1 : Outport
  wires:
  In1/1 -> Out1/1

== system system_2022 [23-03-03]/Subsystem/System Update and Heirarchy/Power_CMD/DC POWER/BAT: >75% ==
  In1 : Inport
  Action Port : ActionPort
  Out1 : Outport
  wires:
  In1/1 -> Out1/1

== system system_2022 [23-03-03]/Subsystem/System Update and Heirarchy/Power_CMD/DC POWER/BAT:>50% ==
  In1 : Inport
  Action Port : ActionPort
  Out1 : Outport
  wires:
  In1/1 -> Out1/1

== system system_2022 [23-03-03]/Subsystem/System Update and Heirarchy/Power_CMD/DC POWER/OUT OF RANGE ==
  In1 : Inport
  Action Port : ActionPort
  Out1 : Outport
  wires:
  In1/1 -> Out1/1

== system system_2022 [23-03-03]/Subsystem/System Update and Heirarchy/Update Internal Variables/Get_HMI_Values/Switch Case Action Subsystem ==
  Value1 : Inport
  Action Port : ActionPort  ActionPortLabel=case [ 0 ]:
  Out1 : Outport
  wires:
  Value1/1 -> Out1/1

== system system_2022 [23-03-03]/Subsystem/System Update and Heirarchy/Update Internal Variables/Get_HMI_Values/Switch Case Action Subsystem1 ==
  Value1 : Inport
  Action Port : ActionPort  ActionPortLabel=case [ 1 ]:
  Out1 : Outport
  wires:
  Value1/1 -> Out1/1

== system system_2022 [23-03-03]/Subsystem/System Update and Heirarchy/Update Internal Variables/Get_HMI_Values/Switch Case Action Subsystem2 ==
  Value1 : Inport
  Action Port : ActionPort  ActionPortLabel=case [ 2 ]:
  Out1 : Outport
  wires:
  Value1/1 -> Out1/1

== system system_2022 [23-03-03]/Subsystem/System Update and Heirarchy/Update Internal Variables/Get_HMI_Values/Switch Case Action Subsystem3 ==
  Value1 : Inport
  Action Port : ActionPort  ActionPortLabel=case [ 3 ]:
  Out1 : Outport
  wires:
  Value1/1 -> Out1/1

== system system_2022 [23-03-03]/Subsystem/System Update and Heirarchy/Update Internal Variables/Get_HMI_Values/Switch Case Action Subsystem4 ==
  Value1 : Inport
  Action Port : ActionPort  ActionPortLabel=case [ 4 ]:
  Out1 : Outport
  wires:
  Value1/1 -> Out1/1

== system system_2022 [23-03-03]/Subsystem/System Update and Heirarchy/Update Internal Variables/Get_HMI_Values/Switch Case Action Subsystem5 ==
  Value1 : Inport
  Action Port : ActionPort  ActionPortLabel=case [ 5 ]:
  Out1 : Outport
  wires:
  Value1/1 -> Out1/1

== system system_2022 [23-03-03]/Subsystem/System Update and Heirarchy/Update Internal Variables/Get_HMI_Values/Switch Case Action Subsystem6 ==
  Value1 : Inport
  Action Port : ActionPort  ActionPortLabel=default:
  Out1 : Outport
  wires:
  Value1/1 -> Out1/1

== system system_2022 [23-03-03]/Subsystem/System Update and Heirarchy/Update Internal Variables/HMI_CMD1/Alarm ==
  note: Alarm I2C_0:
      | Address(0x15)
  note: Alarm Trigger & Disarm
  note: 0x05 (05) - Alarm_Off
      | 0x15 (17) - Alarm_On
  H_Cmd : Inport
  Action Port : ActionPort  ActionPortLabel=case [ 5 ]:
  Alarm_Off : Subsystem  TreatAsAtomicUnit=on
  Data Type Conversion1 : DataTypeConversion  OutDataTypeStr=uint8  SaturateOnIntegerOverflow=off  RndMeth=Floor
  I2C Master Write : mbedblockslib/I2C Master Write  Commented=on  I2CModule=2  Mode=Master  SlaveAddress=uint8(hex2dec('15'))  SlaveByteOrder=BigEndian  Direction=Transmitter  RegisterAddressMode=off  RegisterAddress=uint8(hex2dec('11'))  SlaveDataType=uint8  DataLength=2  NoAck=off  RepeatedStart=off  OutputStatus=off
      settings: SourceProductBaseCode=MICROBIT,NUCLEO,STMICRODIS
  If : If  IfExpression=(u1 == 5)
  Merge : Merge
  START : Subsystem  TreatAsAtomicUnit=on
  dummy : Constant  Value=5
  Elem : Outport
  wires:
  H_Cmd/1 -> If/1
  Merge/1 -> Data Type Conversion1/1
  Alarm_Off/1(Out1) -> Merge/1
  If/2 -> START/Action
  START/1(Out1) -> Merge/2
  dummy/1 -> Elem/1
  If/1 -> Alarm_Off/Action
  Data Type Conversion1/1 -> I2C Master Write/1

== system system_2022 [23-03-03]/Subsystem/System Update and Heirarchy/Update Internal Variables/HMI_CMD1/ERROR MSG ==
  In1 : Inport
  Action Port : ActionPort  ActionPortLabel=default:
  Out1 : Outport
  wires:
  In1/1 -> Out1/1

== system system_2022 [23-03-03]/Subsystem/System Update and Heirarchy/Update Internal Variables/HMI_CMD1/MODE ==
  note: 0x09 (09) - CPAP
      | 0x19 (25) - BiPAP
  note: Mode_0 - CPAP
      | Mode_1 - BiPAP
  H_Cmd : Inport
  Action Port : ActionPort  ActionPortLabel=case [ 9 ]:
  Data Store Write : DataStoreWrite  DataStoreName=Mode  IndexOptions=Index vector (dialog)  Indices=1  OutputSizes=1
  Display : Display
  Element : Constant  Value=5
  If : If  IfExpression=(u1 == 9)
  Merge : Merge
  Mode - BiPAP : Subsystem  TreatAsAtomicUnit=on
  Mode - CPAP : Subsystem  TreatAsAtomicUnit=on
  Elem : Outport
  wires:
  H_Cmd/1 -> If/1
  If/1 -> Mode - CPAP/Action
  If/2 -> Mode - BiPAP/Action
  Merge/1 -> Display/1, Data Store Write/1
  Mode - CPAP/1(Out1) -> Merge/1
  Mode - BiPAP/1(Out1) -> Merge/2
  Element/1 -> Elem/1

== system system_2022 [23-03-03]/Subsystem/System Update and Heirarchy/Update Internal Variables/HMI_CMD1/START ==
  note: 0x01 (01) - START
      | 0x11 (17) - STOP
  H_Cmd : Inport
  Action Port : ActionPort  ActionPortLabel=case [ 1 ]:
  Data Store Write1 : DataStoreWrite  DataStoreName=START  IndexOptions=Index vector (dialog)  Indices=1  OutputSizes=1
  If : If  IfExpression=(u1 == 1)
  Merge : Merge
  START : Subsystem  TreatAsAtomicUnit=on
  STOP : Subsystem  TreatAsAtomicUnit=on
  dummy : Constant  Value=5
  Elem : Outport
  wires:
  START/1(Out1) -> Merge/2
  STOP/1(Out1) -> Merge/1
  Merge/1 -> Data Store Write1/1
  If/2 -> START/Action
  If/1 -> STOP/Action
  H_Cmd/1 -> If/1
  dummy/1 -> Elem/1

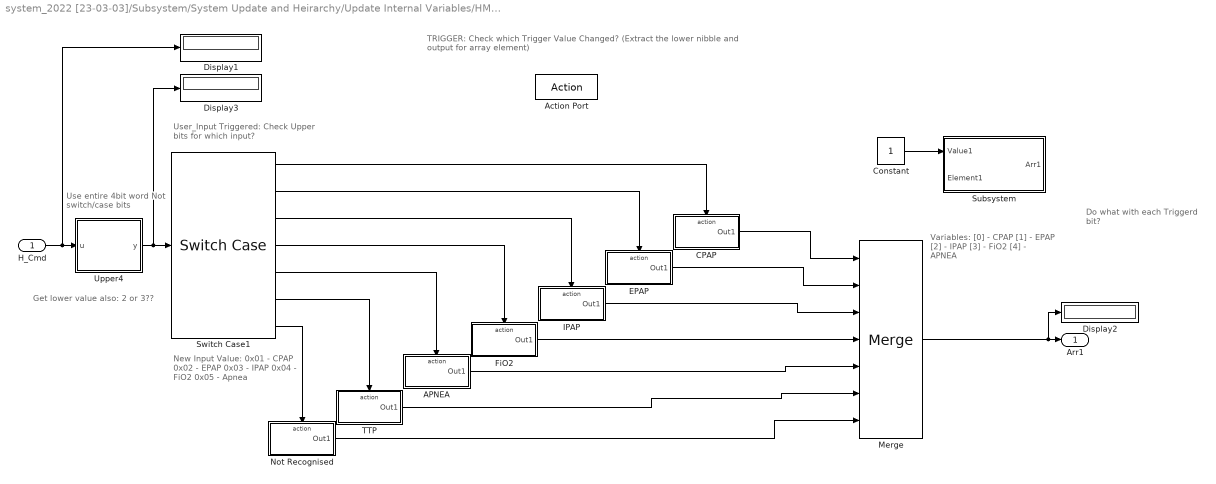
== system system_2022 [23-03-03]/Subsystem/System Update and Heirarchy/Update Internal Variables/HMI_CMD1/User_Input ==
  note: Variables:
      | [0] - CPAP
      | [1] - EPAP
      | [2] - IPAP
      | [3] - FiO2
      | [4] - APNEA
  note: Get lower value also: 2 or 3??
  note: New Input Value:
      | 0x01 - CPAP
      | 0x02 - EPAP
      | 0x03 - IPAP
      | 0x04 - FiO2
      | 0x05 - Apnea
  note: Do what with each
      | Triggerd bit?
  note: Use entire 4bit word
      | Not switch/case bits
  note: User_Input Triggered:
      | Check Upper bits for which input?
  note: TRIGGER: Check which Trigger Value Changed?
      | (Extract the lower nibble and output for array element)
  H_Cmd : Inport
  Action Port : ActionPort  ActionPortLabel=case [ 3 ]:
  APNEA : Subsystem  TreatAsAtomicUnit=on
  CPAP : Subsystem  TreatAsAtomicUnit=on
  Constant : Constant
  Display1 : Display
  Display2 : Display
  Display3 : Display
  EPAP : Subsystem  TreatAsAtomicUnit=on
  FiO2 : Subsystem  TreatAsAtomicUnit=on
  IPAP : Subsystem  TreatAsAtomicUnit=on
  Merge : Merge  Inputs=7
  Not Recognised : Subsystem  TreatAsAtomicUnit=on
  Subsystem : Subsystem
  Switch Case1 : SwitchCase  CaseConditions={0x00, 0x01, 0x02, 0x03, 0x04, 0x05}
  TTP : Subsystem  TreatAsAtomicUnit=on
  Upper4 : Subsystem
  Arr1 : Outport
  wires:
  TTP/1(Out1) -> Merge/6
  APNEA/1(Out1) -> Merge/5
  Merge/1 -> Display2/1, Arr1/1
  Switch Case1/6 -> TTP/Action
  Switch Case1/5 -> APNEA/Action
  Constant/1 -> Subsystem/1(Value1)
  Upper4/1(y) -> Switch Case1/1, Display3/1
  H_Cmd/1 -> Upper4/1(u), Display1/1
  FiO2/1(Out1) -> Merge/4
  IPAP/1(Out1) -> Merge/3
  Switch Case1/4 -> FiO2/Action
  Switch Case1/3 -> IPAP/Action
  Not Recognised/1(Out1) -> Merge/7
  EPAP/1(Out1) -> Merge/2
  CPAP/1(Out1) -> Merge/1
  Switch Case1/7 -> Not Recognised/Action
  Switch Case1/1 -> CPAP/Action
  Switch Case1/2 -> EPAP/Action

== system system_2022 [23-03-03]/Subsystem/System Update and Heirarchy/Update Internal Variables/HMI_CMD1/Alarm/Alarm_Off ==
  note: Alarm(0) = OFF
  Action Port : ActionPort  ActionPortLabel=if((u1 == 5))
  STOP : Constant  Value=0
  Out1 : Outport
  wires:
  STOP/1 -> Out1/1

== system system_2022 [23-03-03]/Subsystem/System Update and Heirarchy/Update Internal Variables/HMI_CMD1/Alarm/START ==
  note: Alarm(1) = ON
  Action Port : ActionPort  ActionPortLabel=else
  START : Constant
  Out1 : Outport
  wires:
  START/1 -> Out1/1

== system system_2022 [23-03-03]/Subsystem/System Update and Heirarchy/Update Internal Variables/HMI_CMD1/MODE/Mode - BiPAP ==
  note: Mode(1) = BiPAP
  Action Port : ActionPort  ActionPortLabel=else
  BiPAP : Constant
  Out1 : Outport
  wires:
  BiPAP/1 -> Out1/1

== system system_2022 [23-03-03]/Subsystem/System Update and Heirarchy/Update Internal Variables/HMI_CMD1/MODE/Mode - CPAP ==
  note: Mode(0) = CPAP
  Action Port : ActionPort  ActionPortLabel=if((u1 == 9))
  CPAP : Constant  Value=0
  Out1 : Outport
  wires:
  CPAP/1 -> Out1/1

== system system_2022 [23-03-03]/Subsystem/System Update and Heirarchy/Update Internal Variables/HMI_CMD1/START/START ==
  note: Mode(1) = BiPAP
  Action Port : ActionPort  ActionPortLabel=else
  START : Constant
  Out1 : Outport
  wires:
  START/1 -> Out1/1

== system system_2022 [23-03-03]/Subsystem/System Update and Heirarchy/Update Internal Variables/HMI_CMD1/START/STOP ==
  note: Mode(0) = CPAP
  Action Port : ActionPort  ActionPortLabel=if((u1 == 1))
  STOP : Constant  Value=0
  Out1 : Outport
  wires:
  STOP/1 -> Out1/1

== system system_2022 [23-03-03]/Subsystem/System Update and Heirarchy/Update Internal Variables/HMI_CMD1/User_Input/APNEA ==
  note: APNEA
  Action Port : ActionPort  ActionPortLabel=case [ 4 ]:
  Constant : Constant  Value=4
  Out1 : Outport
  wires:
  Constant/1 -> Out1/1

== system system_2022 [23-03-03]/Subsystem/System Update and Heirarchy/Update Internal Variables/HMI_CMD1/User_Input/CPAP ==
  Action Port : ActionPort  ActionPortLabel=case [ 0 ]:
  Constant : Constant  Value=0
  Out1 : Outport
  wires:
  Constant/1 -> Out1/1

== system system_2022 [23-03-03]/Subsystem/System Update and Heirarchy/Update Internal Variables/HMI_CMD1/User_Input/EPAP ==
  note: EPAP
  Action Port : ActionPort  ActionPortLabel=case [ 1 ]:
  Constant : Constant
  Out1 : Outport
  wires:
  Constant/1 -> Out1/1

== system system_2022 [23-03-03]/Subsystem/System Update and Heirarchy/Update Internal Variables/HMI_CMD1/User_Input/FiO2 ==
  note: FiO2
  Action Port : ActionPort  ActionPortLabel=case [ 3 ]:
  Constant : Constant  Value=3
  Out1 : Outport
  wires:
  Constant/1 -> Out1/1

== system system_2022 [23-03-03]/Subsystem/System Update and Heirarchy/Update Internal Variables/HMI_CMD1/User_Input/IPAP ==
  note: IPAP
  Action Port : ActionPort  ActionPortLabel=case [ 2 ]:
  Constant : Constant  Value=2
  Out1 : Outport
  wires:
  Constant/1 -> Out1/1

== system system_2022 [23-03-03]/Subsystem/System Update and Heirarchy/Update Internal Variables/HMI_CMD1/User_Input/Not Recognised ==
  note: Must be within array element range [0-3]
  Action Port : ActionPort  ActionPortLabel=default:
  Constant : Constant  Value=0
  Out1 : Outport
  wires:
  Constant/1 -> Out1/1

== system system_2022 [23-03-03]/Subsystem/System Update and Heirarchy/Update Internal Variables/HMI_CMD1/User_Input/Subsystem ==
  note: Update single element of input array
  Value1 : Inport
  Element1 : Inport  Port=2
  Assignment : Assignment  IndexMode=Zero-based  DiagnosticForDimensions=Warning  IndexOptions=Index vector (port)  Indices=0  OutputSizes=1
  Constant5 : Constant  Value=[0,0,0,0]
  Arr1 : Outport
  wires:
  Assignment/1 -> Arr1/1
  Element1/1 -> Assignment/3
  Value1/1 -> Assignment/2
  Constant5/1 -> Assignment/1

== system system_2022 [23-03-03]/Subsystem/System Update and Heirarchy/Update Internal Variables/HMI_CMD1/User_Input/TTP ==
  note: Time To Peak
  Action Port : ActionPort  ActionPortLabel=case [ 5 ]:
  Constant : Constant  Value=5
  Out1 : Outport
  wires:
  Constant/1 -> Out1/1

== system system_2022 [23-03-03]/Subsystem/System Update and Heirarchy/Update Internal Variables/HMI_CMD1/User_Input/Upper4 ==
  note: Get Upper 4 bits
  u : Inport
  Bit Shift1 : hdlsllib/Logic and Bit Operations/Bit Shift  mode=Shift Right Logical  N=4
  Data Type Conversion1 : DataTypeConversion  OutDataTypeStr=uint8  SaturateOnIntegerOverflow=off  RndMeth=Floor
  Extract Bits3 : simulink/Logic and Bit Operations/Extract Bits  bitsToExtract=Upper half  numBits=8  bitIdxRange=[0 7]  outScalingMode=Preserve fixed-point scaling
  y : Outport
  wires:
  u/1 -> Extract Bits3/1
  Extract Bits3/1 -> Data Type Conversion1/1
  Bit Shift1/1 -> y/1
  Data Type Conversion1/1 -> Bit Shift1/1
